simulink model "amplificador_2022b"  (R2022b)
settings: Solver=VariableStepAuto  StartTime=0.0  StopTime=0.003  MaxStep=0.00001  RelTol=1e-3
values from neighbouring files (symbols this model uses):
  alpha1 = beta/(R1*R2*C1*C2)    (= 250000000)    [ampli_int.m]    (also in datos.m)
  gamma1 = (1/(R1*C1))+((1-beta)/(R2*C2))+(1/(R2*C1))    (= 5000)    [ampli_int.m]    (also in datos.m)
  R1 = 1000    [ampli_int.m]    (also in datos.m)
  R2 = 1000    [ampli_int.m]    (also in datos.m)
  R3 = 10000    [ampli_int.m]    (also in datos.m)
  R4 = 15000    [ampli_int.m]    (also in datos.m)
  tau1 = 1/(R1*R2*C1*C2)    (= 100000000)    [ampli_int.m]    (also in datos.m)
libraries: fl_lib x12, nesl_utility x3
settings Model: Creator=mluser  LastModifiedBy=Cris
settings OptimizationCC: ReuseModelBlockBuffer=on

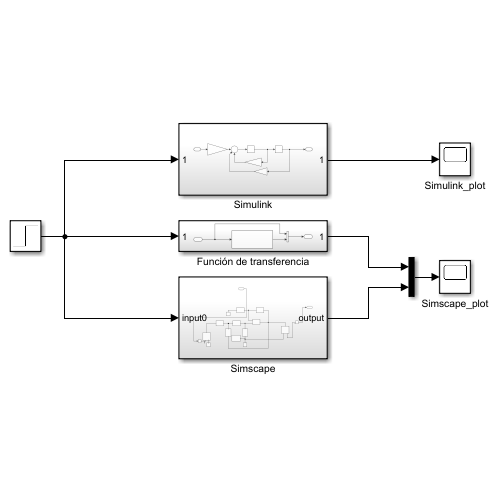
[thumbnail: Simulink's stored preview of the top-level diagram]
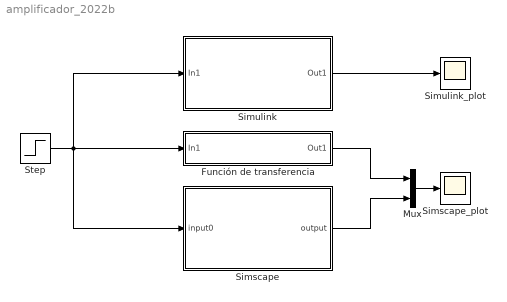
== system amplificador_2022b ==
  Función de transferencia : Subsystem
  Mux : Mux  Inputs=2
  Simscape : Subsystem
  Simscape_plot : Scope
  Simulink : Subsystem
  Simulink_plot : Scope
  Step : Step  Time=0  SampleTime=0
  wires:
  Step/1 -> Simulink/1(In1), Función de transferencia/1(In1), Simscape/1(input0)
  Mux/1 -> Simscape_plot/1
  Función de transferencia/1(Out1) -> Mux/1
  Simscape/1(output) -> Mux/2
  Simulink/1(Out1) -> Simulink_plot/1

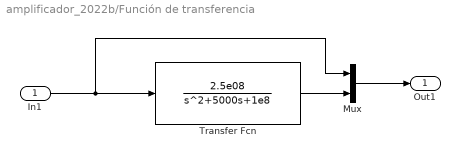
== system amplificador_2022b/Función de transferencia ==
  In1 : Inport
  Mux : Mux  Inputs=2
  Transfer Fcn : TransferFcn  Numerator=2.5e08  Denominator=[1 5000 1e8]
  Out1 : Outport
  wires:
  In1/1 -> Mux/1, Transfer Fcn/1
  Mux/1 -> Out1/1
  Transfer Fcn/1 -> Mux/2

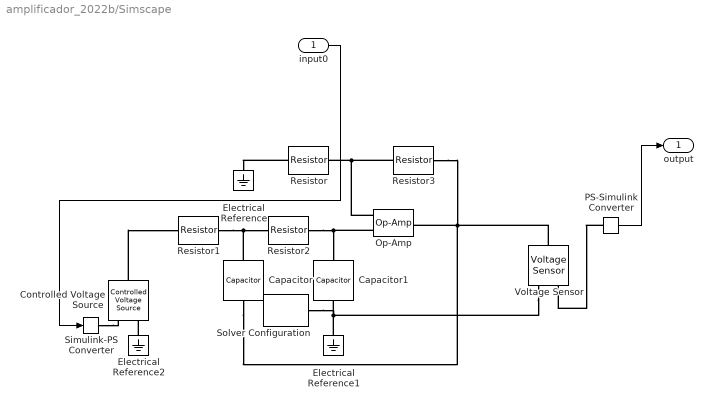
== system amplificador_2022b/Simscape ==
  input0 : Inport
  Capacitor : fl_lib/Electrical/Electrical Elements/Capacitor  c=C1 F  r=1e-6 Ohm  g=0 1/Ohm  i_specify=off  i_priority=None  i=0 A  i_nominal_specify=off  i_nominal_unit=A  i_nominal_value=1  v_specify=off  v_priority=None  v=0 V  v_nominal_specify=off  v_nominal_unit=V  v_nominal_value=1  vc_specify=off  vc_priority=High  vc=0 V  vc_nominal_specify=off  vc_nominal_unit=V  vc_nominal_value=1
  Capacitor1 : fl_lib/Electrical/Electrical Elements/Capacitor  c=C2 F  r=1e-6 Ohm  g=0 1/Ohm  i_specify=off  i_priority=None  i=0 A  i_nominal_specify=off  i_nominal_unit=A  i_nominal_value=1  v_specify=off  v_priority=None  v=0 V  v_nominal_specify=off  v_nominal_unit=V  v_nominal_value=1  vc_specify=off  vc_priority=High  vc=0 V  vc_nominal_specify=off  vc_nominal_unit=V  vc_nominal_value=1
  Controlled Voltage Source : fl_lib/Electrical/Electrical Sources/Controlled Voltage Source
  Electrical Reference : fl_lib/Electrical/Electrical Elements/Electrical Reference
  Electrical Reference1 : fl_lib/Electrical/Electrical Elements/Electrical Reference
  Electrical Reference2 : fl_lib/Electrical/Electrical Elements/Electrical Reference
  Op-Amp : fl_lib/Electrical/Electrical Elements/Op-Amp  outI_specify=off  outI_priority=None  outI=0 A  outI_nominal_specify=off  outI_nominal_unit=A  outI_nominal_value=1
  PS-Simulink Converter : nesl_utility/PS-Simulink Converter  PhysicalDomain=network_engine_domain  SubClassName=ps_output  LeftPortType=input  RightPortType=output  PseudoPeriodic=off  Frequencies=[]  VectorFormat=inherit  Unit=inherit  AffineConversion=off
  Resistor : fl_lib/Electrical/Electrical Elements/Resistor  R=R3 Ohm  i_specify=off  i_priority=None  i=0 A  i_nominal_specify=off  i_nominal_unit=A  i_nominal_value=1  v_specify=off  v_priority=None  v=0 V  v_nominal_specify=off  v_nominal_unit=V  v_nominal_value=1
  Resistor1 : fl_lib/Electrical/Electrical Elements/Resistor  R=R1 Ohm  i_specify=off  i_priority=None  i=0 A  i_nominal_specify=off  i_nominal_unit=A  i_nominal_value=1  v_specify=off  v_priority=None  v=0 V  v_nominal_specify=off  v_nominal_unit=V  v_nominal_value=1
  Resistor2 : fl_lib/Electrical/Electrical Elements/Resistor  R=R2 Ohm  i_specify=off  i_priority=None  i=0 A  i_nominal_specify=off  i_nominal_unit=A  i_nominal_value=1  v_specify=off  v_priority=None  v=0 V  v_nominal_specify=off  v_nominal_unit=V  v_nominal_value=1
  Resistor3 : fl_lib/Electrical/Electrical Elements/Resistor  R=R4 Ohm  i_specify=off  i_priority=None  i=0 A  i_nominal_specify=off  i_nominal_unit=A  i_nominal_value=1  v_specify=off  v_priority=None  v=0 V  v_nominal_specify=off  v_nominal_unit=V  v_nominal_value=1
  Simulink-PS Converter : nesl_utility/Simulink-PS Converter  PhysicalDomain=network_engine_domain  SubClassName=ps_input  LeftPortType=input  RightPortType=output  PseudoPeriodic=off  Frequencies=[]  NoiseDistribution=none  NoiseParameters=[]  Unit=1  AffineConversion=off  FilteringAndDerivatives=provide  SimscapeFilterOrder=1  InputFilterTimeConstant=0.001  UdotUserProvided=0
  Solver Configuration : nesl_utility/Solver Configuration  PhysicalDomain=network_engine_domain  SubClassName=solver  LeftPortType=input  RightPortType=generic  Tones=[]  Harmonics=[]  SimulateNoise=off  Profile=off  UseLocalSampling=off  EnableSwitchedLinearOptims=on  FrequencyDomain=off  UseCCode=off  RelTol=0.001  AbsTol=0.001  MinStep=1e-09  ToWorkspace=off  RevertToSquareIcSolve=off  NumHomotopyIterations=100  PhasorMode=off  PhasorModeNumHarmonics=1  ConsistencySolver=NEWTON_XTOL_AFTER_FTOL  IndexReductionMethod=DerivativeReplacement  DoDC=off  ResidualTolerance=1e-09  ConsistencyTolSource=GLOBAL  ConsistencyAbsTol=0.001  ConsistencyRelTol=0.001  ConsistencyTolFactor=0.001  UseLocalSolver=off  LocalSolverChoice=NE_BACKWARD_EULER_ADVANCER  ResolveIndetEquations=on  FunctionEvalNumThread=1  LocalSolverSampleTime=0.001  DoFixedCost=off  MaxNonlinIter=3  MaxModeIter=2  ComputeImpulses=off  ImpulseIterations=2  LinearAlgebra=auto  LinearAlgebraNumThread=0  EquationFormulation=NE_TIME_EF  DelaysMemoryBudget=1024  AutomaticFiltering=on  FilteringTimeConstant=0.001  PartitionStorageMethod=AS_NEEDED  PartitionMemoryBudget=1024  PartitionMethod=ROBUST
  Voltage Sensor : fl_lib/Electrical/Electrical Sensors/Voltage Sensor
  output : Outport
  wires:
  input0/1 -> Simulink-PS Converter/1
  PS-Simulink Converter/1 -> output/1
  connections:
  Controlled Voltage Source/LConn1 -- Resistor1/LConn1
  Resistor/LConn1 -- Electrical Reference/LConn1
  Electrical Reference2/LConn1 -- Controlled Voltage Source/RConn2
  Simulink-PS Converter/RConn1 -- Controlled Voltage Source/RConn1
  Electrical Reference1/LConn1 -- Capacitor1/RConn1 -- Solver Configuration/RConn1 -- Voltage Sensor/RConn2
  PS-Simulink Converter/LConn1 -- Voltage Sensor/RConn1
  Capacitor/LConn1 -- Resistor1/RConn1 -- Resistor2/LConn1
  Resistor3/RConn1 -- Capacitor/RConn1 -- Voltage Sensor/LConn1 -- Op-Amp/RConn1
  Op-Amp/LConn1 -- Resistor/RConn1 -- Resistor3/LConn1
  Resistor2/RConn1 -- Capacitor1/LConn1 -- Op-Amp/LConn2

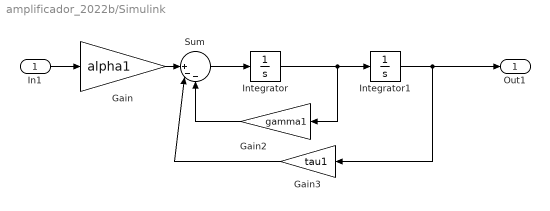
== system amplificador_2022b/Simulink ==
  In1 : Inport
  Gain : Gain  Gain=alpha1
  Gain2 : Gain  Gain=gamma1
  Gain3 : Gain  Gain=tau1
  Integrator : Integrator
  Integrator1 : Integrator
  Sum : Sum  Inputs=||+--
  Out1 : Outport
  wires:
  Integrator/1 -> Integrator1/1, Gain2/1
  Integrator1/1 -> Out1/1, Gain3/1
  In1/1 -> Gain/1
  Gain2/1 -> Sum/3
  Gain3/1 -> Sum/2
  Gain/1 -> Sum/1
  Sum/1 -> Integrator/1
